simulink model "basicINS"  (R2015a)
settings: Solver=FixedStepDiscrete  StartTime=0.0  StopTime=100  RelTol=1e-3
PreLoadFcn:
  | load INSdata.mat
InitFcn:
  | InitNav;
  | dtSensor = inertialData_ts.angular_rate.Time(2)-inertialData_ts.angular_rate.Time(1);
values from neighbouring files (symbols this model uses):
  centripetalL = [0;0;0]    [InitNav.m]
  coriolisL = [0;0;0]    [InitNav.m]
  earthRateL = [0;0;0]    [InitNav.m]
  gravityL = -[0;0;earthConstants.gStd]    [InitNav.m]
  inertialData_ts =     [INSdataHoneywell.mat]
  initialAltitude = 147.882    [InitNav.m]
  initialHeading = 0    [InitNav.m]
  initialLatitude = 34.042872 * convert.degTorad    [InitNav.m]
  initialLongitude = 118.696816 * convert.degTorad    [InitNav.m]
  initialPitch = 0    [InitNav.m]
  initialRoll = 0    [InitNav.m]
  initialVelocityL = [0;0;0]    [InitNav.m]
  initialYaw = 0    [InitNav.m]
  t_initialize = tS    (= 0.001)    [InitNav.m]
  transportRateL = [0;0;0]    [InitNav.m]
  tS = 1/fS    (= 0.001)    [InitNav.m]
undefined symbols (not defined in the file or in its folder): earthConstants, earthRadii, NavData
libraries: simulink_extras x16, vrlib x3
settings Model: SimulationMode=accelerator  Creator=dlwalter  LastModifiedBy=dlwalter
settings DataIOCC: SignalLoggingSaveFormat=ModelDataLogs
settings OptimizationCC: BlockReduction=off  ConditionallyExecuteInputs=off  ExpressionDepthLimit=2147483647
settings DebuggingCC: SolverPrmCheckMsg=warning  FcnCallInpInsideContextMsg=EnableAllAsWarning  StateNameClashWarn=warning

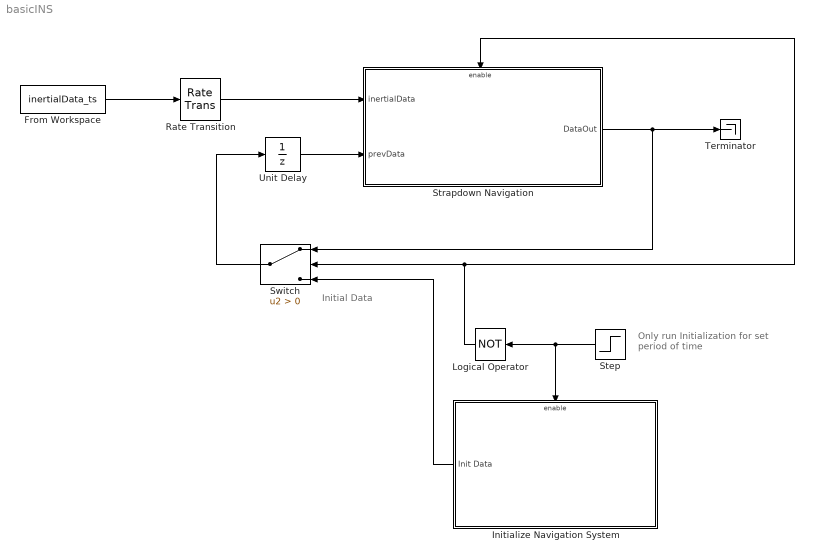
== system basicINS ==
  note: Only run Initialization
      |  for set period of time
  note: Initial Data
  From Workspace : FromWorkspace  VariableName=inertialData_ts  OutDataTypeStr=Bus: BInertialData  SampleTime=0  OutputAfterFinalValue=Holding final value
  Initialize Navigation System : Subsystem  TreatAsAtomicUnit=on
  Logical Operator : Logic  Operator=NOT  AllPortsSameDT=off  OutDataTypeStr=boolean
  Rate Transition : RateTransition  OutPortSampleTime=tS
  Step : Step  Time=t_initialize  Before=1  After=0  SampleTime=tS
  Strapdown Navigation : Subsystem
  Switch : Switch  Criteria=u2 > Threshold
  Terminator : Terminator
  Unit Delay : UnitDelay  SampleTime=-1
  wires:
  From Workspace/1 -> Rate Transition/1
  Rate Transition/1 -> Strapdown Navigation/1(inertialData)
  Initialize Navigation System/1(Init Data) -> Switch/3
  Logical Operator/1 -> Switch/2, Strapdown Navigation/Enable
  Switch/1 -> Unit Delay/1
  Step/1 -> Logical Operator/1, Initialize Navigation System/Enable
  Unit Delay/1 -> Strapdown Navigation/2(prevData)
  Strapdown Navigation/1(DataOut) -> Switch/1, Terminator/1

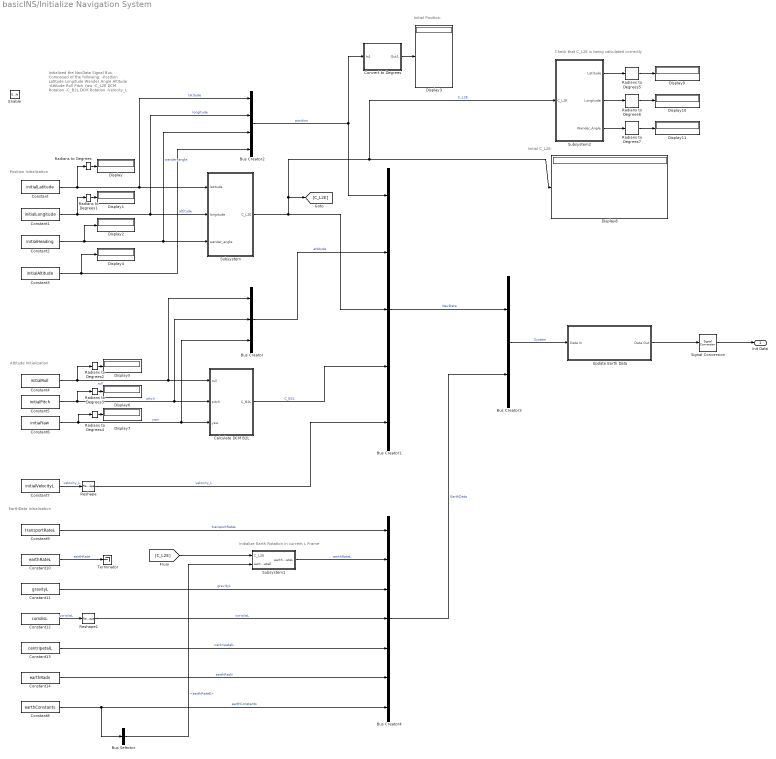
== system basicINS/Initialize Navigation System ==
  note: Check that C_L2E is being calculated correctly
  note: Initial C_L2E:
  note: Initial Position:
  note: Initialize Earth Rotation in current L Frame
  note: EarthData Initialization
  note: Attitude Initialization
  note: Position Initialization
  note: Initialized the NavData Signal Bus.
      | Composed of the following:
      | 	-Position
      | 		Latitude
      | 		Longitude
      | 		Wander Angle
      | 		Altitude
      | 	-Attitude
      | 		Roll
      | 		Pitch
      | 		Yaw
      | 	-C_L2E DCM Rotation
      | 	-C_B2L DCM Rotation
      | 	-Velocity_L
  Enable : EnablePort
  Bus Creator : BusCreator  Inputs=3  OutDataTypeStr=Bus: BAttitude
  Bus Creator1 : BusCreator  Inputs='position','attitude','C_L2E','C_B2L','velocity_L'  OutDataTypeStr=Bus: BNavData
  Bus Creator2 : BusCreator  OutDataTypeStr=Bus: BPosition
  Bus Creator3 : BusCreator  Inputs='NavData','EarthData'
  Bus Creator4 : BusCreator  Inputs=7
  Bus Selector : BusSelector  OutputSignals=earthRateE
  Calculate DCM B2L : Subsystem
  Constant : Constant  Value=initialLatitude
  Constant1 : Constant  Value=initialLongitude
  Constant10 : Constant  Value=earthRateL
  Constant11 : Constant  Value=gravityL
  Constant12 : Constant  Value=coriolisL
  Constant13 : Constant  Value=centripetalL
  Constant14 : Constant  Value=earthRadii  OutDataTypeStr=Bus: BEarthRadii
  Constant2 : Constant  Value=initialHeading
  Constant3 : Constant  Value=initialAltitude
  Constant4 : Constant  Value=initialRoll
  Constant5 : Constant  Value=initialPitch
  Constant6 : Constant  Value=initialYaw
  Constant7 : Constant  Value=initialVelocityL
  Constant8 : Constant  Value=earthConstants  OutDataTypeStr=Bus: BEarthConstants
  Constant9 : Constant  Value=transportRateL
  Convert to Degrees : Subsystem
  Display{,1..11} (12 alike) : Display
  Radians to Degrees{,1..7} (8 alike) : simulink_extras/Transformations/Radians to Degrees
  Reshape : Reshape  OutputDimensionality=Column vector (2-D)
  Reshape1 : Reshape  OutputDimensionality=Column vector (2-D)
  Signal Conversion : SignalConversion
  Subsystem : Subsystem
  Subsystem1 : Subsystem
  Subsystem2 : Subsystem
  Terminator : Terminator
  Update Earth Data : Subsystem
  Init Data : Outport  OutDataTypeStr=Bus: BSystem
  wires:
  Constant/1 -> Bus Creator2/1, Subsystem/1(latitude), Radians to Degrees/1  "latitude"
  Constant1/1 -> Bus Creator2/2, Subsystem/2(longitude), Radians to Degrees1/1  "longitude"
  Constant2/1 -> Display2/1, Bus Creator2/3, Subsystem/3(wander_angle)  "wander_angle"
  Constant3/1 -> Display4/1, Bus Creator2/4  "altitude"
  Constant7/1 -> Reshape/1  "velocity_L"
  Bus Creator2/1 -> Convert to Degrees/1(In1), Bus Creator1/1  "position"
  Bus Creator/1 -> Bus Creator1/2  "attitude"
  Subsystem/1(C_L2E) -> Subsystem2/1(C_L2E), Display8/1, [C_L2E], Bus Creator1/3  "C_L2E"
  Calculate DCM B2L/1(C_B2L) -> Bus Creator1/4  "C_B2L"
  Bus Creator1/1 -> Bus Creator3/1  "NavData"
  Constant14/1 -> Bus Creator4/6  "earthRadii"
  Constant12/1 -> Reshape1/1  "coriolisL"
  Constant9/1 -> Bus Creator4/1  "transportRateL"
  Constant11/1 -> Bus Creator4/3  "gravityL"
  Constant13/1 -> Bus Creator4/5  "centripetalL"
  Bus Creator4/1 -> Bus Creator3/2  "EarthData"
  Constant8/1 -> Bus Selector/1, Bus Creator4/7  "earthConstants"
  Subsystem1/1(earthRateL) -> Bus Creator4/2  "earthRateL"
  Bus Selector/1 -> Subsystem1/2(earthRateE)  "<earthRateE>"
  [C_L2E] -> Subsystem1/1(C_L2E)
  Constant10/1 -> Terminator/1  "earthRate"
  Reshape/1 -> Bus Creator1/5  "velocity_L"
  Reshape1/1 -> Bus Creator4/4  "coriolisL"
  Bus Creator3/1 -> Update Earth Data/1(Data In)  "System"
  Convert to Degrees/1(Out1) -> Display3/1
  Update Earth Data/1(Data Out) -> Signal Conversion/1
  Signal Conversion/1 -> Init Data/1
  Radians to Degrees/1 -> Display/1
  Radians to Degrees1/1 -> Display1/1
  Constant4/1 -> Radians to Degrees2/1, Bus Creator/1, Calculate DCM B2L/1(roll)  "roll"
  Radians to Degrees2/1 -> Display5/1
  Constant5/1 -> Radians to Degrees3/1, Calculate DCM B2L/2(pitch), Bus Creator/2  "pitch"
  Radians to Degrees3/1 -> Display6/1
  Constant6/1 -> Calculate DCM B2L/3(yaw), Bus Creator/3, Radians to Degrees4/1  "yaw"
  Radians to Degrees4/1 -> Display7/1
  Subsystem2/1(Latitude) -> Radians to Degrees5/1
  Radians to Degrees5/1 -> Display9/1
  Subsystem2/2(Longitude) -> Radians to Degrees6/1
  Radians to Degrees6/1 -> Display10/1
  Subsystem2/3(Wander_Angle) -> Radians to Degrees7/1
  Radians to Degrees7/1 -> Display11/1

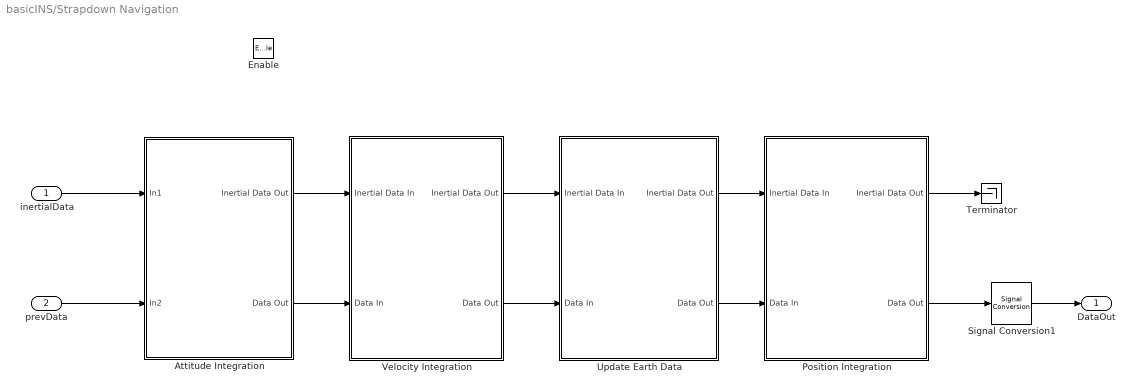
== system basicINS/Strapdown Navigation ==
  inertialData : Inport
  prevData : Inport  Port=2  OutDataTypeStr=Bus: BSystem
  Enable : EnablePort
  Attitude Integration : Subsystem
  Position Integration : Subsystem
  Signal Conversion1 : SignalConversion
  Terminator : Terminator
  Update Earth Data : Subsystem
  Velocity Integration : Subsystem
  DataOut : Outport  OutDataTypeStr=Bus: BSystem
  wires:
  inertialData/1 -> Attitude Integration/1(In1)
  prevData/1 -> Attitude Integration/2(In2)
  Attitude Integration/2(Data Out) -> Velocity Integration/2(Data In)
  Attitude Integration/1(Inertial Data Out) -> Velocity Integration/1(Inertial Data In)
  Velocity Integration/1(Inertial Data Out) -> Update Earth Data/1(Inertial Data In)
  Velocity Integration/2(Data Out) -> Update Earth Data/2(Data In)
  Update Earth Data/1(Inertial Data Out) -> Position Integration/1(Inertial Data In)
  Update Earth Data/2(Data Out) -> Position Integration/2(Data In)
  Position Integration/1(Inertial Data Out) -> Terminator/1
  Position Integration/2(Data Out) -> Signal Conversion1/1
  Signal Conversion1/1 -> DataOut/1

== system basicINS/Initialize Navigation System/Calculate DCM B2L ==
  note: Computes DCM Rotational Matrix
      | from Body Frame to Earth Frame
  roll : Inport
  pitch : Inport  Port=2
  yaw : Inport  Port=3
  MATLAB Function : MATLAB Function  TreatAsAtomicUnit=on
  C_B2L : Outport
  wires:
  MATLAB Function/1(C_B2L) -> C_B2L/1
  roll/1 -> MATLAB Function/1(roll)
  pitch/1 -> MATLAB Function/2(pitch)
  yaw/1 -> MATLAB Function/3(yaw)

== system basicINS/Initialize Navigation System/Convert to Degrees ==
  In1 : Inport
  Bus Creator3 : BusCreator  OutDataTypeStr=Bus: BPosition
  Bus Selector4 : BusSelector  OutputSignals=latitude,longitude,wander_angle,altitude
  Radians to Degrees : simulink_extras/Transformations/Radians to Degrees
  Radians to Degrees1 : simulink_extras/Transformations/Radians to Degrees
  Out1 : Outport
  wires:
  Radians to Degrees/1 -> Bus Creator3/1  "latitude"
  Bus Selector4/1 -> Radians to Degrees/1  "<latitude>"
  Bus Selector4/2 -> Radians to Degrees1/1  "<longitude>"
  Bus Selector4/3 -> Bus Creator3/3  "<wander_angle>"
  Radians to Degrees1/1 -> Bus Creator3/2  "longitude"
  Bus Selector4/4 -> Bus Creator3/4  "<altitude>"
  In1/1 -> Bus Selector4/1
  Bus Creator3/1 -> Out1/1

== system basicINS/Initialize Navigation System/Subsystem ==
  note: Computes DCM Rotation Matrix
      | from Local Frame to Earth Frame
  latitude : Inport
  longitude : Inport  Port=2
  wander_angle : Inport  Port=3
  MATLAB Function : MATLAB Function  TreatAsAtomicUnit=on
  C_L2E : Outport
  wires:
  MATLAB Function/1(C_L2E) -> C_L2E/1
  latitude/1 -> MATLAB Function/1(lat)
  longitude/1 -> MATLAB Function/2(long)
  wander_angle/1 -> MATLAB Function/3(wander)

== system basicINS/Initialize Navigation System/Subsystem1 ==
  C_L2E : Inport
  earthRateE : Inport  Port=2
  Math Function : Math  Operator=transpose  SaturateOnIntegerOverflow=on
  Product : Product  Multiplication=Matrix(*)
  earthRateL : Outport
  wires:
  C_L2E/1 -> Math Function/1
  Product/1 -> earthRateL/1  "earthRateL"
  earthRateE/1 -> Product/2
  Math Function/1 -> Product/1  "C_E2L"

== system basicINS/Initialize Navigation System/Subsystem2 ==
  C_L2E : Inport
  MATLAB Function : MATLAB Function  TreatAsAtomicUnit=on
  Latitude : Outport
  Longitude : Outport  Port=2
  Wander_Angle : Outport  Port=3
  wires:
  C_L2E/1 -> MATLAB Function/1(cL2E)
  MATLAB Function/3(wan) -> Wander_Angle/1
  MATLAB Function/2(lon) -> Longitude/1
  MATLAB Function/1(lat) -> Latitude/1

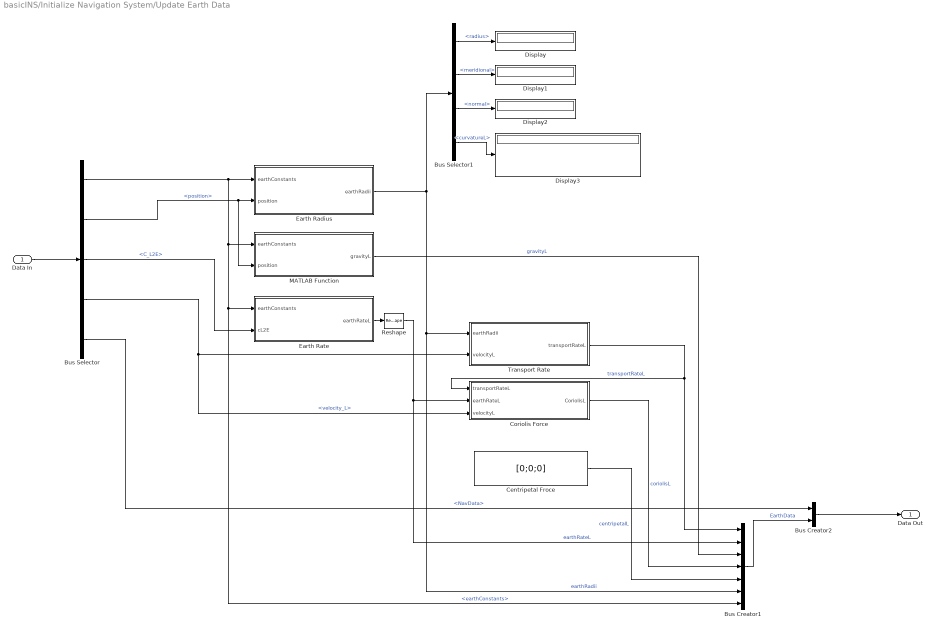
== system basicINS/Initialize Navigation System/Update Earth Data ==
  Data In : Inport
  Bus Creator1 : BusCreator  Inputs=7  OutDataTypeStr=Bus: BEarthData
  Bus Creator2 : BusCreator  Inputs=2  OutDataTypeStr=Bus: BSystem
  Bus Selector : BusSelector  OutputSignals=EarthData.earthConstants,NavData.position,NavData.C_L2E,NavData.velocity_L,NavData
  Bus Selector1 : BusSelector  OutputSignals=radius,meridional,normal,curvatureL
  Centripetal Froce : Constant  Value=[0;0;0]
  Coriolis Force : Subsystem
  Display{,1..3} (4 alike) : Display
  "Earth Radius " : MATLAB Function  TreatAsAtomicUnit=on
  Earth Rate : MATLAB Function  TreatAsAtomicUnit=on
  MATLAB Function : MATLAB Function  TreatAsAtomicUnit=on
  Reshape : Reshape  OutputDimensionality=Column vector (2-D)
  Transport Rate : MATLAB Function  TreatAsAtomicUnit=on
  Data Out : Outport  OutDataTypeStr=Bus: BSystem
  wires:
  Data In/1 -> Bus Selector/1
  Bus Selector/1 -> Bus Creator1/7, Earth Rate/1(earthConstants), MATLAB Function/1(earthConstants), "Earth Radius "/1(earthConstants)  "<earthConstants>"
  Bus Selector/2 -> MATLAB Function/2(position), "Earth Radius "/2(position)  "<position>"
  Bus Selector/3 -> Earth Rate/2(cL2E)  "<C_L2E>"
  Bus Selector/4 -> Coriolis Force/3(velocityL), Transport Rate/2(velocityL)  "<velocity_L>"
  Bus Creator1/1 -> Bus Creator2/2  "EarthData"
  Bus Selector/5 -> Bus Creator2/1  "<NavData>"
  "Earth Radius "/1(earthRadii) -> Bus Selector1/1, Bus Creator1/6, Transport Rate/1(earthRadii)  "earthRadii"
  Transport Rate/1(transportRateL) -> Bus Creator1/1, Coriolis Force/1(transportRateL)  "transportRateL"
  Bus Creator2/1 -> Data Out/1
  Centripetal Froce/1 -> Bus Creator1/5  "centripetalL"
  Coriolis Force/1(CoriolisL) -> Bus Creator1/4  "coriolisL"
  Earth Rate/1(earthRateL) -> Reshape/1
  MATLAB Function/1(gravityL) -> Bus Creator1/3  "gravityL"
  Reshape/1 -> Coriolis Force/2(earthRateL), Bus Creator1/2  "earthRateL"
  Bus Selector1/1 -> Display/1  "<radius>"
  Bus Selector1/2 -> Display1/1  "<meridional>"
  Bus Selector1/3 -> Display2/1  "<normal>"
  Bus Selector1/4 -> Display3/1  "<curvatureL>"

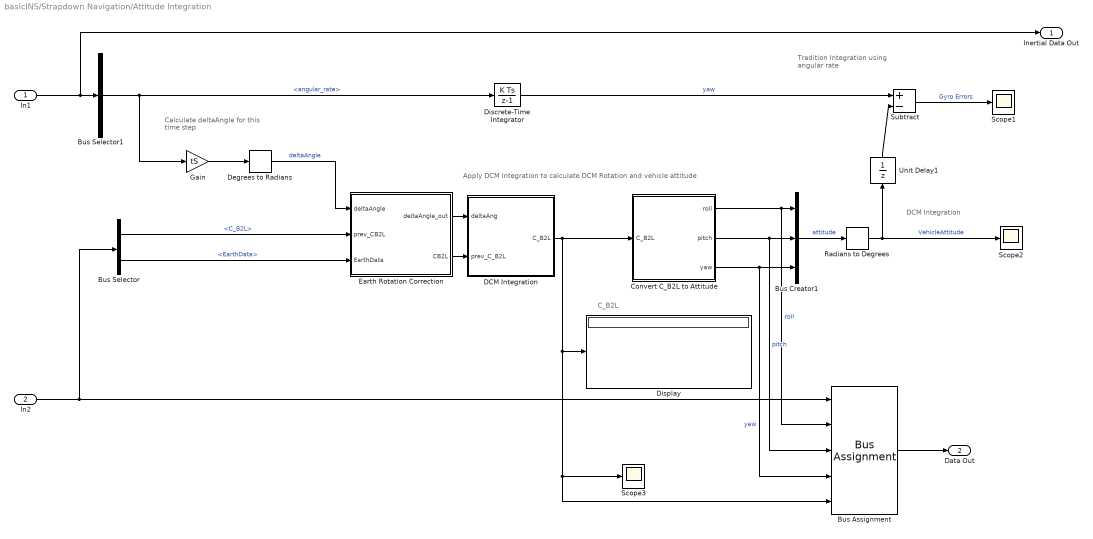
== system basicINS/Strapdown Navigation/Attitude Integration ==
  note: C_B2L
  note: Apply DCM Integration to calculate DCM Rotation and vehicle attitude
  note: DCM Integration
  note: Tradition Integration
      | using angular rate
  note: Calculate deltaAngle
      | for this time step
  In1 : Inport
  In2 : Inport  Port=2
  Bus Assignment : BusAssignment  AssignedSignals=NavData.attitude.roll,NavData.attitude.pitch,NavData.attitude.yaw,NavData.C_B2L
  Bus Creator1 : BusCreator  Inputs=3
  Bus Selector : BusSelector  OutputSignals=NavData.C_B2L,EarthData
  Bus Selector1 : BusSelector  OutputSignals=angular_rate
  Convert C_B2L to Attitude : Subsystem
  DCM Integration : Subsystem
  Degrees to Radians : simulink_extras/Transformations/Degrees to Radians
  Discrete-Time Integrator : DiscreteIntegrator  SampleTime=tS
  Display : Display
  Earth Rotation Correction : Subsystem
  Gain : Gain  Gain=tS
  Radians to Degrees : simulink_extras/Transformations/Radians to Degrees
  Scope1 : Scope
      settings: ShowLegends=on  SaveName=gyroErrors
  Scope2 : Scope
      settings: YMin=-0.25  YMax=2.5  SaveName=ScopeData2
  Scope3 : Scope
  Subtract : Sum  Inputs=+-
  Unit Delay1 : UnitDelay  SampleTime=-1
  Inertial Data Out : Outport
  Data Out : Outport  Port=2
  wires:
  Bus Selector/1 -> Earth Rotation Correction/2(prev_CB2L)  "<C_B2L>"
  Earth Rotation Correction/2(CB2L) -> DCM Integration/2(prev_C_B2L)
  Degrees to Radians/1 -> Earth Rotation Correction/1(deltaAngle)  "deltaAngle"
  Earth Rotation Correction/1(deltaAngle_out) -> DCM Integration/1(deltaAng)
  Bus Selector1/1 -> Gain/1, Discrete-Time Integrator/1  "<angular_rate>"
  Discrete-Time Integrator/1 -> Subtract/1  "yaw"
  In1/1 -> Inertial Data Out/1, Bus Selector1/1
  Gain/1 -> Degrees to Radians/1
  Convert C_B2L to Attitude/1(roll) -> Bus Assignment/2, Bus Creator1/1  "roll"
  Convert C_B2L to Attitude/2(pitch) -> Bus Assignment/3, Bus Creator1/2  "pitch"
  Convert C_B2L to Attitude/3(yaw) -> Bus Assignment/4, Bus Creator1/3  "yaw"
  Bus Creator1/1 -> Radians to Degrees/1  "attitude"
  Radians to Degrees/1 -> Scope2/1, Unit Delay1/1  "VehicleAttitude"
  Bus Selector/2 -> Earth Rotation Correction/3(EarthData)  "<EarthData>"
  In2/1 -> Bus Assignment/1, Bus Selector/1
  Unit Delay1/1 -> Subtract/2
  Subtract/1 -> Scope1/1  "Gyro Errors"
  Bus Assignment/1 -> Data Out/1
  DCM Integration/1(C_B2L) -> Convert C_B2L to Attitude/1(C_B2L), Display/1, Scope3/1, Bus Assignment/5

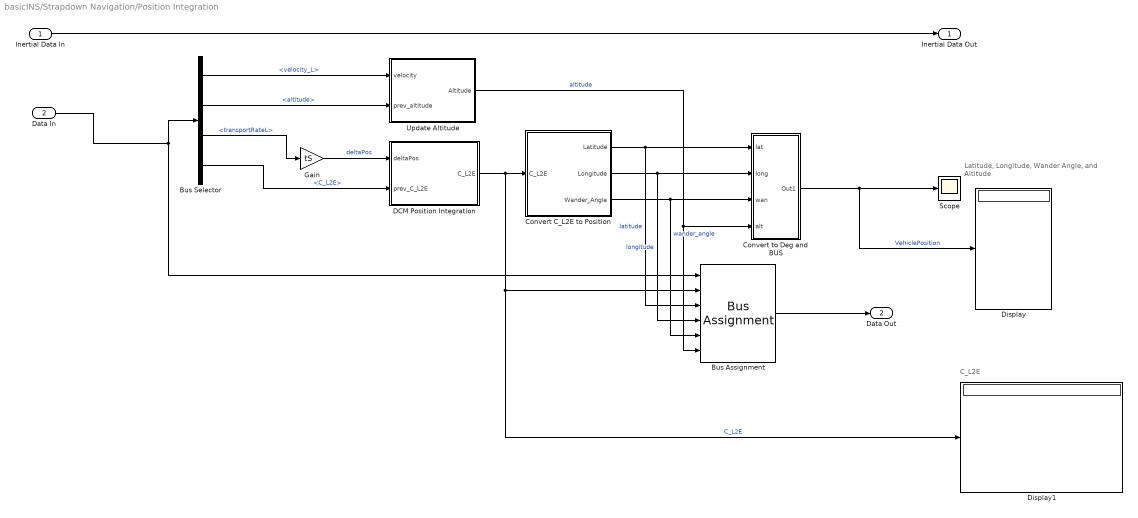
== system basicINS/Strapdown Navigation/Position Integration ==
  note: C_L2E
  note: Latitude, Longitude, Wander Angle,
      | and Altitude
  Inertial Data In : Inport
  Data In : Inport  Port=2
  Bus Assignment : BusAssignment  AssignedSignals=NavData.C_L2E,NavData.position.latitude,NavData.position.longitude,NavData.position.wander_angle,NavData.position.altitude
  Bus Selector : BusSelector  OutputSignals=NavData.velocity_L,NavData.position.altitude,EarthData.transportRateL,NavData.C_L2E
  Convert C_L2E to Position : Subsystem
  Convert to Deg and BUS : Subsystem
  DCM Position Integration : Subsystem
  Display : Display
  Display1 : Display
  Gain : Gain  Gain=tS
  Scope : Scope
      settings: ShowLegends=on  YMin=-250  YMax=1750  SaveName=ScopeData9
  Update Altitude : Subsystem
  Inertial Data Out : Outport
  Data Out : Outport  Port=2
  wires:
  Data In/1 -> Bus Assignment/1, Bus Selector/1
  Inertial Data In/1 -> Inertial Data Out/1
  DCM Position Integration/1(C_L2E) -> Convert C_L2E to Position/1(C_L2E), Display1/1, Bus Assignment/2  "C_L2E"
  Gain/1 -> DCM Position Integration/1(deltaPos)  "deltaPos"
  Convert C_L2E to Position/1(Latitude) -> Bus Assignment/3, Convert to Deg and BUS/1(lat)  "latitude"
  Convert C_L2E to Position/2(Longitude) -> Convert to Deg and BUS/2(long), Bus Assignment/4  "longitude"
  Update Altitude/1(Altitude) -> Bus Assignment/6, Convert to Deg and BUS/4(alt)  "altitude"
  Bus Assignment/1 -> Data Out/1
  Bus Selector/1 -> Update Altitude/1(velocity)  "<velocity_L>"
  Bus Selector/2 -> Update Altitude/2(prev_altitude)  "<altitude>"
  Bus Selector/4 -> DCM Position Integration/2(prev_C_L2E)  "<C_L2E>"
  Bus Selector/3 -> Gain/1  "<transportRateL>"
  Convert C_L2E to Position/3(Wander_Angle) -> Convert to Deg and BUS/3(wan), Bus Assignment/5  "wander_angle"
  Convert to Deg and BUS/1(Out1) -> Display/1, Scope/1  "VehiclePosition"

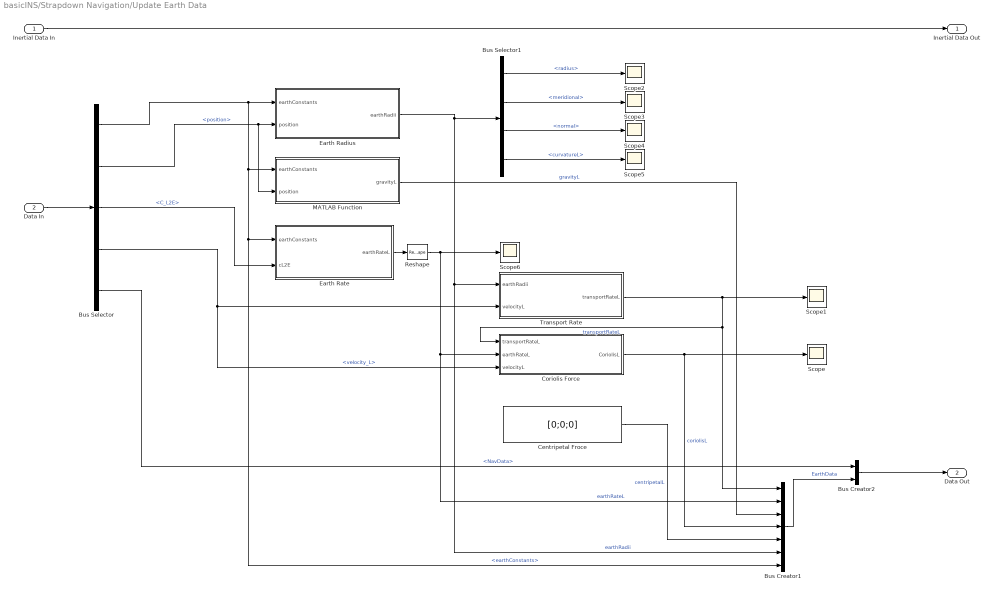
== system basicINS/Strapdown Navigation/Update Earth Data ==
  Inertial Data In : Inport
  Data In : Inport  Port=2
  Bus Creator1 : BusCreator  Inputs=7  OutDataTypeStr=Bus: BEarthData
  Bus Creator2 : BusCreator  Inputs=2  OutDataTypeStr=Bus: BSystem
  Bus Selector : BusSelector  OutputSignals=EarthData.earthConstants,NavData.position,NavData.C_L2E,NavData.velocity_L,NavData
  Bus Selector1 : BusSelector  OutputSignals=radius,meridional,normal,curvatureL
  Centripetal Froce : Constant  Value=[0;0;0]
  Coriolis Force : Subsystem
  "Earth Radius " : MATLAB Function  TreatAsAtomicUnit=on
  Earth Rate : MATLAB Function  TreatAsAtomicUnit=on
  MATLAB Function : MATLAB Function  TreatAsAtomicUnit=on
  Reshape : Reshape  OutputDimensionality=Column vector (2-D)
  Scope{,1..6} (7 alike) : Scope
      Scope settings: ShowLegends=on  SaveName=ScopeData4
      Scope1 settings: ShowLegends=on  SaveName=ScopeData6
      Scope2 settings: SaveName=ScopeData10
      Scope3 settings: SaveName=ScopeData11
      Scope4 settings: SaveName=ScopeData12
      Scope5 settings: SaveName=ScopeData13
      Scope6 settings: ShowLegends=on  SaveName=ScopeData17
  Transport Rate : MATLAB Function  TreatAsAtomicUnit=on
  Inertial Data Out : Outport
  Data Out : Outport  Port=2  OutDataTypeStr=Bus: BSystem
  wires:
  Inertial Data In/1 -> Inertial Data Out/1
  Data In/1 -> Bus Selector/1
  Bus Selector/1 -> Bus Creator1/7, Earth Rate/1(earthConstants), MATLAB Function/1(earthConstants), "Earth Radius "/1(earthConstants)  "<earthConstants>"
  Bus Selector/2 -> MATLAB Function/2(position), "Earth Radius "/2(position)  "<position>"
  Bus Selector/3 -> Earth Rate/2(cL2E)  "<C_L2E>"
  Bus Selector/4 -> Coriolis Force/3(velocityL), Transport Rate/2(velocityL)  "<velocity_L>"
  Bus Creator1/1 -> Bus Creator2/2  "EarthData"
  Bus Selector/5 -> Bus Creator2/1  "<NavData>"
  "Earth Radius "/1(earthRadii) -> Bus Creator1/6, Transport Rate/1(earthRadii), Bus Selector1/1  "earthRadii"
  Transport Rate/1(transportRateL) -> Scope1/1, Bus Creator1/1, Coriolis Force/1(transportRateL)  "transportRateL"
  Bus Creator2/1 -> Data Out/1
  Centripetal Froce/1 -> Bus Creator1/5  "centripetalL"
  Coriolis Force/1(CoriolisL) -> Bus Creator1/4, Scope/1  "coriolisL"
  Earth Rate/1(earthRateL) -> Reshape/1
  MATLAB Function/1(gravityL) -> Bus Creator1/3  "gravityL"
  Reshape/1 -> Scope6/1, Coriolis Force/2(earthRateL), Bus Creator1/2  "earthRateL"
  Bus Selector1/4 -> Scope5/1  "<curvatureL>"
  Bus Selector1/1 -> Scope2/1  "<radius>"
  Bus Selector1/2 -> Scope3/1  "<meridional>"
  Bus Selector1/3 -> Scope4/1  "<normal>"

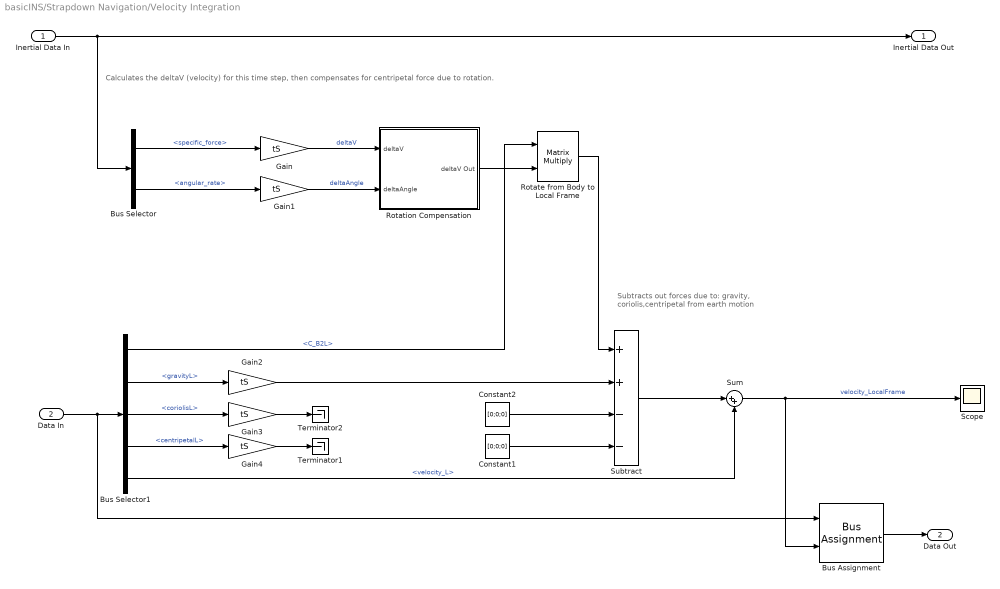
== system basicINS/Strapdown Navigation/Velocity Integration ==
  note: Subtracts out forces due to:
      | gravity, coriolis,centripetal from earth motion
  note: Calculates the deltaV (velocity) for this time step, then compensates for centripetal force due to rotation.
  Inertial Data In : Inport
  Data In : Inport  Port=2
  Bus Assignment : BusAssignment  AssignedSignals=NavData.velocity_L
  Bus Selector : BusSelector  OutputSignals=specific_force,angular_rate
  Bus Selector1 : BusSelector  OutputSignals=NavData.C_B2L,EarthData.gravityL,EarthData.coriolisL,EarthData.centripetalL,NavData.velocity_L
  Constant1 : Constant  Value=[0;0;0]
  Constant2 : Constant  Value=[0;0;0]
  Gain{,1..4} (5 alike) : Gain  Gain=tS
  Rotate from Body to Local Frame : Product  Multiplication=Matrix(*)
  Rotation Compensation : Subsystem
  Scope : Scope
      settings: ShowLegends=on  YMin=-150  YMax=150
  Subtract : Sum  Inputs=++--
  Sum : Sum  Inputs=|++
  Terminator1 : Terminator
  Terminator2 : Terminator
  Inertial Data Out : Outport
  Data Out : Outport  Port=2  OutDataTypeStr=Bus: BSystem
  wires:
  Inertial Data In/1 -> Bus Selector/1, Inertial Data Out/1
  Bus Selector/1 -> Gain/1  "<specific_force>"
  Bus Selector/2 -> Gain1/1  "<angular_rate>"
  Gain/1 -> Rotation Compensation/1(deltaV)  "deltaV"
  Gain1/1 -> Rotation Compensation/2(deltaAngle)  "deltaAngle"
  Bus Selector1/1 -> Rotate from Body to Local Frame/1  "<C_B2L>"
  Rotation Compensation/1(deltaV Out) -> Rotate from Body to Local Frame/2
  Bus Selector1/2 -> Gain2/1  "<gravityL>"
  Bus Selector1/3 -> Gain3/1  "<coriolisL>"
  Bus Selector1/4 -> Gain4/1  "<centripetalL>"
  Gain2/1 -> Subtract/2
  Rotate from Body to Local Frame/1 -> Subtract/1
  Subtract/1 -> Sum/1
  Bus Selector1/5 -> Sum/2  "<velocity_L>"
  Sum/1 -> Bus Assignment/2, Scope/1  "velocity_LocalFrame"
  Data In/1 -> Bus Assignment/1, Bus Selector1/1
  Bus Assignment/1 -> Data Out/1
  Gain4/1 -> Terminator1/1
  Constant1/1 -> Subtract/4
  Constant2/1 -> Subtract/3
  Gain3/1 -> Terminator2/1

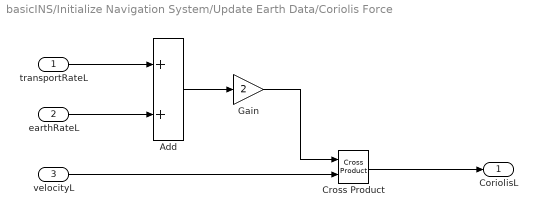
== system basicINS/Initialize Navigation System/Update Earth Data/Coriolis Force ==
  transportRateL : Inport
  earthRateL : Inport  Port=2
  velocityL : Inport  Port=3
  Add : Sum
  Cross Product : vrlib/Utilities/Cross Product
  Gain : Gain  Gain=2
  CoriolisL : Outport
  wires:
  transportRateL/1 -> Add/1
  earthRateL/1 -> Add/2
  Add/1 -> Gain/1
  Cross Product/1 -> CoriolisL/1
  Gain/1 -> Cross Product/1
  velocityL/1 -> Cross Product/2

== system basicINS/Strapdown Navigation/Attitude Integration/Convert C_B2L to Attitude ==
  C_B2L : Inport
  MATLAB Function : MATLAB Function  TreatAsAtomicUnit=on
  roll : Outport
  pitch : Outport  Port=2
  yaw : Outport  Port=3
  wires:
  C_B2L/1 -> MATLAB Function/1(cB2L)
  MATLAB Function/1(rol) -> roll/1
  MATLAB Function/2(pch) -> pitch/1
  MATLAB Function/3(yaw) -> yaw/1

== system basicINS/Strapdown Navigation/Attitude Integration/DCM Integration ==
  deltaAng : Inport
  prev_C_B2L : Inport  Port=2
  MATLAB Function : MATLAB Function  TreatAsAtomicUnit=on
  C_B2L : Outport
  wires:
  prev_C_B2L/1 -> MATLAB Function/2(cPastX2Y)
  deltaAng/1 -> MATLAB Function/1(dXp2Xn)
  MATLAB Function/1(cOutX2Y) -> C_B2L/1

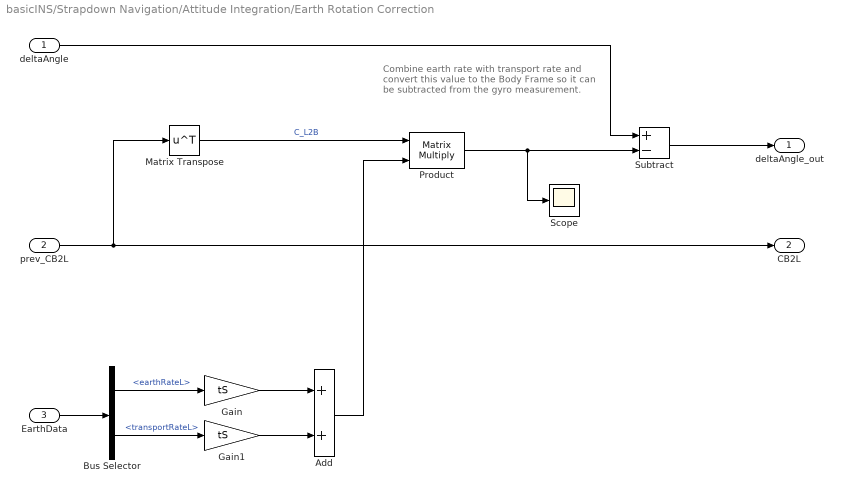
== system basicINS/Strapdown Navigation/Attitude Integration/Earth Rotation Correction ==
  note: Combine earth rate with transport rate
      | and convert this value to the Body Frame
      | so it can be subtracted from the gyro
      | measurement.
  deltaAngle : Inport
  prev_CB2L : Inport  Port=2
  EarthData : Inport  Port=3
  Add : Sum
  Bus Selector : BusSelector  OutputSignals=earthRateL,transportRateL
  Gain : Gain  Gain=tS
  Gain1 : Gain  Gain=tS
  Matrix Transpose : Math  Operator=transpose  SaturateOnIntegerOverflow=on
  Product : Product  Multiplication=Matrix(*)
  Scope : Scope
      settings: YMin=-5e-08  YMax=7e-08  SaveName=ScopeData3
  Subtract : Sum  Inputs=+-
  deltaAngle_out : Outport
  CB2L : Outport  Port=2
  wires:
  prev_CB2L/1 -> Matrix Transpose/1, CB2L/1
  EarthData/1 -> Bus Selector/1
  Bus Selector/1 -> Gain/1  "<earthRateL>"
  Bus Selector/2 -> Gain1/1  "<transportRateL>"
  Gain/1 -> Add/1
  deltaAngle/1 -> Subtract/1
  Matrix Transpose/1 -> Product/1  "C_L2B"
  Add/1 -> Product/2
  Subtract/1 -> deltaAngle_out/1
  Gain1/1 -> Add/2
  Product/1 -> Scope/1, Subtract/2

== system basicINS/Strapdown Navigation/Position Integration/Convert C_L2E to Position ==
  C_L2E : Inport
  MATLAB Function1 : MATLAB Function  TreatAsAtomicUnit=on
  Latitude : Outport
  Longitude : Outport  Port=2
  Wander_Angle : Outport  Port=3
  wires:
  C_L2E/1 -> MATLAB Function1/1(cL2E)
  MATLAB Function1/3(wan) -> Wander_Angle/1
  MATLAB Function1/2(lon) -> Longitude/1
  MATLAB Function1/1(lat) -> Latitude/1

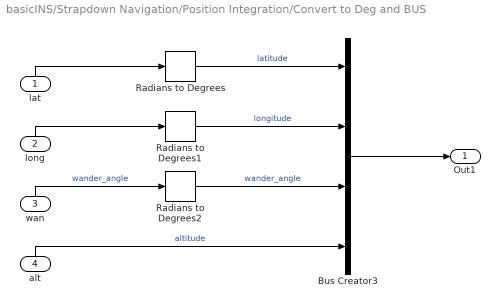
== system basicINS/Strapdown Navigation/Position Integration/Convert to Deg and BUS ==
  lat : Inport
  long : Inport  Port=2
  wan : Inport  Port=3
  alt : Inport  Port=4
  Bus Creator3 : BusCreator  OutDataTypeStr=Bus: BPosition
  Radians to Degrees : simulink_extras/Transformations/Radians to Degrees
  Radians to Degrees1 : simulink_extras/Transformations/Radians to Degrees
  Radians to Degrees2 : simulink_extras/Transformations/Radians to Degrees
  Out1 : Outport
  wires:
  Radians to Degrees1/1 -> Bus Creator3/2  "longitude"
  Radians to Degrees/1 -> Bus Creator3/1  "latitude"
  Bus Creator3/1 -> Out1/1
  lat/1 -> Radians to Degrees/1
  long/1 -> Radians to Degrees1/1
  wan/1 -> Radians to Degrees2/1  "wander_angle"
  alt/1 -> Bus Creator3/4  "altitude"
  Radians to Degrees2/1 -> Bus Creator3/3  "wander_angle"

== system basicINS/Strapdown Navigation/Position Integration/DCM Position Integration ==
  deltaPos : Inport
  prev_C_L2E : Inport  Port=2
  MATLAB Function : MATLAB Function  TreatAsAtomicUnit=on
  C_L2E : Outport
  wires:
  prev_C_L2E/1 -> MATLAB Function/2(cPastX2Y)
  deltaPos/1 -> MATLAB Function/1(dXp2Xn)
  MATLAB Function/1(cOutX2Y) -> C_L2E/1

== system basicINS/Strapdown Navigation/Position Integration/Update Altitude ==
  note: Note: +vL(z) is -delta Altitude
  velocity : Inport
  prev_altitude : Inport  Port=2
  Gain : Gain  Gain=tS
  Selector : Selector  InputPortWidth=3  Indices=[3]
  Sum1 : Sum  Inputs=|++
  Altitude : Outport
  wires:
  Gain/1 -> Sum1/2  "deltaH"
  Selector/1 -> Gain/1
  velocity/1 -> Selector/1
  Sum1/1 -> Altitude/1
  prev_altitude/1 -> Sum1/1

== system basicINS/Strapdown Navigation/Update Earth Data/Coriolis Force ==
  transportRateL : Inport
  earthRateL : Inport  Port=2
  velocityL : Inport  Port=3
  Add : Sum
  Cross Product : vrlib/Utilities/Cross Product
  Gain : Gain  Gain=2
  CoriolisL : Outport
  wires:
  transportRateL/1 -> Add/1
  earthRateL/1 -> Add/2
  Add/1 -> Gain/1
  Cross Product/1 -> CoriolisL/1
  Gain/1 -> Cross Product/1
  velocityL/1 -> Cross Product/2

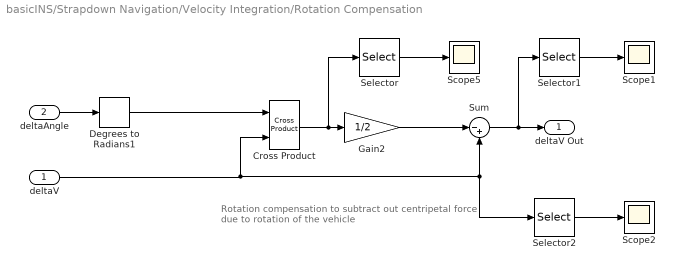
== system basicINS/Strapdown Navigation/Velocity Integration/Rotation Compensation ==
  note: Rotation compensation to subtract out centripetal
      | force due to rotation of the vehicle
  deltaV : Inport
  deltaAngle : Inport  Port=2
  Cross Product : vrlib/Utilities/Cross Product
  Degrees to Radians1 : simulink_extras/Transformations/Degrees to Radians
  Gain2 : Gain  Gain=1/2
  Scope1 : Scope
      settings: ShowLegends=on  SaveName=ScopeData8
  Scope2 : Scope
      settings: ShowLegends=on  SaveName=ScopeData18
  Scope5 : Scope
      settings: ShowLegends=on  SaveName=ScopeData7
  Selector : Selector  InputPortWidth=3  Indices=[2]
  Selector1 : Selector  InputPortWidth=3  Indices=[2]
  Selector2 : Selector  InputPortWidth=3  Indices=[2]
  Sum : Sum  Inputs=|-+
  deltaV Out : Outport
  wires:
  Cross Product/1 -> Selector/1, Gain2/1
  Degrees to Radians1/1 -> Cross Product/1
  Gain2/1 -> Sum/1
  Sum/1 -> deltaV Out/1, Selector1/1
  deltaAngle/1 -> Degrees to Radians1/1
  deltaV/1 -> Selector2/1, Sum/2, Cross Product/2
  Selector/1 -> Scope5/1
  Selector1/1 -> Scope1/1
  Selector2/1 -> Scope2/1

== matlab function basicINS/Initialize Navigation System/Subsystem/MATLAB Function ==
  data: lat input; C_L2E output; long input; wander input
function C_L2E  = DCM_L2E(lat, long, wander)
    
    % Calculate DCM Rotation C_E2L:
   
    align_axes =   [0 0 1;...
                    0 1 0;...
                   -1 0 0];

    Rotate_wander = [cos(wander)   sin(wander) 0; ...
                    -sin(wander)   cos(wander) 0; ...
                    0               0          1];
    
    %Transpose on Latitude term since positive latitude change is a
    %negative rotation about Y Earth axis
    
    Rotate_lat =  [cos(lat) 0        sin(lat);...
                   0        1         0;...
                   -sin(lat) 0         cos(lat)];
    
   Rotate_long  = [1           0           0; ...
                    0   cos(long)   sin(long); ...
                    0  -sin(long)    cos(long)];   
       
    %C_L2E = C_E2L'

    C_L2E = ( Rotate_wander * Rotate_lat * Rotate_long * align_axes )';

== matlab function basicINS/Initialize Navigation System/Calculate DCM B2L/MATLAB Function ==
  data: roll input; C_B2L output; pitch input; yaw input
function C_B2L = DCM_B2L(roll, pitch, yaw)


    Rotate_roll = [1        0                   0; ...
                   0        cos(roll)   sin(roll); ...
                   0       -sin(roll)   cos(roll)];

    Rotate_pitch =[cos(pitch) 0        -sin(pitch);...
                   0          1         0;...
                   sin(pitch) 0         cos(pitch)];
    
    Rotate_yaw  = [cos(yaw)   sin(yaw)  0;...
                  -sin(yaw)   cos(yaw)  0;...
                   0          0         1];
               

    C_B2L = Rotate_roll * Rotate_pitch * Rotate_yaw;

== matlab function basicINS/Strapdown Navigation/Update Earth Data/Earth Radius  ==
  data: earthConstants input; earthRadii output Bus: BEarthRadii; position input
function earthRadii   = Radii(earthConstants, position)
%#codegen

r = zeros(3,1);

earthRadii.radius          = 0;
earthRadii.meridional      = 0;
earthRadii.normal          = 0;


t1 = (earthConstants.radiusEquator^2*cos(position.latitude))^2 + (earthConstants.radiusPolar^2*sin(position.latitude))^2;  % convenience computation
t2 = (earthConstants.radiusEquator*cos(position.latitude))^2 + (earthConstants.radiusPolar*sin(position.latitude))^2;     % convenience computation

% Wikipedia - http://en.wikipedia.org/wiki/Earth_radius
earthRadii.radius     = position.altitude + sqrt(t1/t2);                      % radius at a geodetic latitude
earthRadii.meridional = position.altitude + (earthConstants.radiusEquator * earthConstants.radiusPolar)^2 / (t2)^1.5; % Meridian, radius of curvature
earthRadii.normal     = position.altitude +  earthConstants.radiusEquator^2            / (t2)^0.5; % Normal, radius of curvature

%% Compute the approximate radius of curvature for 
%  local level.
aa = earthRadii.meridional;
bb = earthRadii.normal;
r(1) = aa*bb / sqrt( (bb*cos(position.wander_angle     ))^2 + (aa*sin(position.wander_angle     ))^2);
r(2) = aa*bb / sqrt( (bb*cos(position.wander_angle+pi/2))^2 + (aa*sin(position.wander_angle+pi/2))^2);
    
earthRadii.curvatureL = [       0      1/r(2)      0;   ...
                             -1/r(1)    0          0;   ...
                                0       0          0      ];

== matlab function basicINS/Strapdown Navigation/Update Earth Data/Earth Rate ==
  data: earthConstants input; earthRateL output; cL2E input
function earthRateL = EarthRate(earthConstants, cL2E)
%#codegen

persistent earthRatePastL;

if isempty(earthRatePastL)
    %earthRatePastL = zeros(3,1);
    earthRatePastL = cL2E' * earthConstants.earthRateE;
    %
end
earthRateI = earthConstants.earthRateE;

earthRateInstantL = cL2E' * earthConstants.earthRateE;

earthRateL = (earthRateInstantL + earthRatePastL) / 2;

earthRatePastL = earthRateInstantL;

== matlab function basicINS/Strapdown Navigation/Update Earth Data/MATLAB Function ==
  data: earthConstants input; gravityL output; position input
function gravityL = Gravity(earthConstants,position)
%#codegen


sin2Lat = sin(position.latitude)^2;
h       = position.altitude;
a       = earthConstants.radiusEquator;
b       = earthConstants.radiusPolar;
e       = earthConstants.e;
f       = earthConstants.f;
gm      = earthConstants.gm;
k       = ((b * earthConstants.gPolar)/(a*earthConstants.gEquator))-1;
m       = earthConstants.earthRateE(3)^2 * a^2 * b / gm;

gNormal = earthConstants.gEquator * ...
          (1 + k * sin2Lat) / ...
          sqrt(1 - e^2 * sin2Lat);

t1 = (2 / a) * (1 + f + m - 2 * f * sin2Lat) * h;
t2 = (3 / a^2) * h^2;
gAltitude = gNormal * ( 1 - t1 + t2 );

gravityE = -[0; 0; gAltitude];
gravityL =  gravityE;  % E and L gravity are the 
                       % same since the Z axis of the E and L frames
                       % are colinear

== matlab function basicINS/Strapdown Navigation/Update Earth Data/Transport Rate ==
  data: earthRadii input; transportRateL output; velocityL input
function transportRateL  = TransportRate(earthRadii,velocityL)
%#codegen

persistent vPastL;

if isempty(vPastL)
    %vPastL = zeros(3,1);
    vPastL = velocityL;
end

vAvgL = (vPastL + velocityL) / 2;
transportRateL = earthRadii.curvatureL * vAvgL;

vPastL = velocityL;

== matlab function basicINS/Initialize Navigation System/Update Earth Data/Earth Radius  ==
  data: earthConstants input; earthRadii output Bus: BEarthRadii; position input
function earthRadii   = Radii(earthConstants, position)
%#codegen




r = zeros(3,1);

earthRadii.radius          = 0;
earthRadii.meridional      = 0;
earthRadii.normal          = 0;


t1 = (earthConstants.radiusEquator^2*cos(position.latitude))^2 + (earthConstants.radiusPolar^2*sin(position.latitude))^2;  % convenience computation
t2 = (earthConstants.radiusEquator*cos(position.latitude))^2 + (earthConstants.radiusPolar*sin(position.latitude))^2;     % convenience computation

% Wikipedia - http://en.wikipedia.org/wiki/Earth_radius
earthRadii.radius     = position.altitude + sqrt(t1/t2);                      % radius at a geodetic latitude
earthRadii.meridional = position.altitude + (earthConstants.radiusEquator * earthConstants.radiusPolar)^2 / (t2)^1.5; % Meridian, radius of curvature
earthRadii.normal     = position.altitude +  earthConstants.radiusEquator^2            / (t2)^0.5; % Normal, radius of curvature

%% Compute the approximate radius of curvature for 
%  local level.
aa = earthRadii.meridional;
bb = earthRadii.normal;
r(1) = aa*bb / sqrt( (bb*cos(position.wander_angle     ))^2 + (aa*sin(position.wander_angle     ))^2);
r(2) = aa*bb / sqrt( (bb*cos(position.wander_angle+pi/2))^2 + (aa*sin(position.wander_angle+pi/2))^2);
    
earthRadii.curvatureL = [       0      1/r(2)      0;   ...
                             -1/r(1)    0          0;   ...
                                0       0          0      ];

== matlab function basicINS/Initialize Navigation System/Update Earth Data/Earth Rate ==
  data: earthConstants input; earthRateL output; cL2E input
function earthRateL = EarthRate(earthConstants, cL2E)
%#codegen

persistent earthRatePastL;

if isempty(earthRatePastL)
    earthRatePastL = zeros(3,1);
end

earthRateInstantL = cL2E' * earthConstants.earthRateE;

earthRateL = (earthRateInstantL + earthRatePastL) / 2;

earthRatePastL = earthRateInstantL;

== matlab function basicINS/Initialize Navigation System/Update Earth Data/MATLAB Function ==
  data: earthConstants input; gravityL output; position input
function gravityL = Gravity(earthConstants,position)
%#codegen


sin2Lat = sin(position.latitude)^2;
h       = position.altitude;
a       = earthConstants.radiusEquator;
b       = earthConstants.radiusPolar;
e       = earthConstants.e;
f       = earthConstants.f;
gm      = earthConstants.gm;
k       = ((b * earthConstants.gPolar)/(a*earthConstants.gEquator))-1;
m       = earthConstants.earthRateE(3)^2 * a^2 * b / gm;

gNormal = earthConstants.gEquator * ...
          (1 + k * sin2Lat) / ...
          sqrt(1 - e^2 * sin2Lat);

t1 = (2 / a) * (1 + f + m - 2 * f * sin2Lat) * h;
t2 = (3 / a^2) * h^2;
gAltitude = gNormal * ( 1 - t1 + t2 );

gravityE = -[0; 0; gAltitude];
gravityL =  gravityE;  % E and L gravity are the 
                       % same since the Z axis of the E and L frames
                       % are colinear

== matlab function basicINS/Initialize Navigation System/Update Earth Data/Transport Rate ==
  data: earthRadii input; transportRateL output; velocityL input
function transportRateL  = TransportRate(earthRadii,velocityL)
%#codegen

persistent vPastL;

if isempty(vPastL)
    %vPastL = zeros(3,1);
    vPastL = velocityL;
end

vAvgL = (vPastL + velocityL) / 2;
transportRateL = earthRadii.curvatureL * vAvgL;

vPastL = velocityL;

== matlab function basicINS/Strapdown Navigation/Position Integration/DCM Position Integration/MATLAB Function ==
  data: dXp2Xn input; cOutX2Y output; cPastX2Y input
function cOutX2Y = DcmIntegration(dXp2Xn,cPastX2Y)
%#codegen


    i        = eye(3,3);
    mag      = norm(dXp2Xn);
    drSs     = MySkewSym(dXp2Xn);

    if mag < 1e-04
        cOutX2Y = cPastX2Y * (i+drSs);
    else
        % out = in * (I + sin(mag)/mag * [angle X] + (1-cos(mag) / mag^2 * [angle X]^2;

        t1 = sin(mag)/mag * drSs;
        t2 = (1 - cos(mag)) / mag.^2 * drSs * drSs;

        cBp2Bn = i + t1 + t2;

        cOutX2Y = cPastX2Y * cBp2Bn;
    end


cOutX2Y = [cOutX2Y(:,1)/norm(cOutX2Y (:,1)) ...
          cOutX2Y(:,2)/norm(cOutX2Y(:,2)) cOutX2Y(:,3)/norm(cOutX2Y (:,3))];
    

end

function      out = MySkewSym(in)

    out = zeros(3,3);

    out(1,1) =  0.0;   out(1,2) = -in(3);   out(1,3) =  in(2);
    out(2,1)=  in(3);  out(2,2) =  0.0;     out(2,3) = -in(1);
    out(3,1)= -in(2);  out(3,2) =  in(1);   out(3,3) =  0.0;
end

== matlab function basicINS/Strapdown Navigation/Attitude Integration/DCM Integration/MATLAB Function ==
  data: dXp2Xn input; cOutX2Y output; cPastX2Y input
function cOutX2Y = DcmIntegration(dXp2Xn,cPastX2Y)
%#codegen


    i        = eye(3,3);
    mag      = norm(dXp2Xn);
    drSs     = MySkewSym(dXp2Xn);

    if mag < 1e-04
        cOutX2Y = cPastX2Y * (i+drSs);
    else
        % out = in * (I + sin(mag)/mag * [angle X] + (1-cos(mag) / mag^2 * [angle X]^2;

        t1 = sin(mag)/mag * drSs;
        t2 = (1 - cos(mag)) / mag.^2 * drSs * drSs;

        cBp2Bn = i + t1 + t2;

        cOutX2Y = cPastX2Y * cBp2Bn;
    end
    
    cOutX2Y = [cOutX2Y(:,1)/norm(cOutX2Y (:,1)) ...
          cOutX2Y(:,2)/norm(cOutX2Y(:,2)) cOutX2Y(:,3)/norm(cOutX2Y (:,3))];
    
    %{
    % Should ortho normalize, but for now just limit all elements to 
    % less than 1
    for i=1:3
        for j=1:3
            if cOutX2Y(i,j) > 1
                cOutX2Y(i,j) = 1.0;
            elseif cOutX2Y(i,j) < -1
               cOutX2Y(i,j) = -1.0;
            end
        end
    end
    %}

end

function      out = MySkewSym(in)

    out = zeros(3,3);

    out(1,1) =  0.0;   out(1,2) = -in(3);   out(1,3) =  in(2);
    out(2,1)=  in(3);  out(2,2) =  0.0;     out(2,3) = -in(1);
    out(3,1)= -in(2);  out(3,2) =  in(1);   out(3,3) =  0.0;
end

== matlab function basicINS/Strapdown Navigation/Attitude Integration/Convert C_B2L to Attitude/MATLAB Function ==
  data: cB2L input; rol output; pch output; yaw output
function [rol, pch, yaw]  = EulFromDcmB2L(cB2L)
%#codegen



% limit DCM elements when close to zero
if abs(cB2L(3,3)) < 1e-6
    t1 = 1e-6;
else
    t1 = cB2L(3,3);
end

if abs(cB2L(1,1)) < 1e-6
    t2 = 1e-6;
else
    t2 = cB2L(1,1);
end


rol = atan2(cB2L(3,2),t1);
pch = asin(-cB2L(3,1));
yaw = atan2(cB2L(2,1),t2);

== matlab function basicINS/Initialize Navigation System/Subsystem2/MATLAB Function ==
  data: lat output; cL2E input; lon output; wan output
function [lat, lon, wan]  = LlaFromDcmL2E(cL2E)
%#codegen

%cE2L = cL2E';
lon = atan2(-cL2E(2,3),-cL2E(1,3));
lat = asin (-cL2E(3,3));
wan = atan2(-cL2E(3,2),cL2E(3,1));
%lon = atan2(-cE2L(3,2),-cE2L(3,1));
%lat = -asin(cE2L(3,3));
%wan = atan2(-cE2L(2,3), cE2L(1,3));

== matlab function basicINS/Strapdown Navigation/Position Integration/Convert C_L2E to Position/MATLAB Function1 ==
  data: lat output; cL2E input; lon output; wan output
function [lat, lon, wan]  = LlaFromDcmL2E(cL2E)
%#codegen

%cE2L = cL2E';
lon = atan2(-cL2E(2,3),-cL2E(1,3));
lat = asin (-cL2E(3,3));
wan = atan2(-cL2E(3,2),cL2E(3,1));
%lon = atan2(-cE2L(3,2),-cE2L(3,1));
%lat = -asin(cE2L(3,3));
%wan = atan2(-cE2L(2,3), cE2L(1,3));
